simulink model "testcontroller"  (R2024b)
settings: Solver=VariableStepAuto  StartTime=0.0  StopTime=100.0  RelTol=1e-3
undefined symbols (not defined in the file): f, LF
libraries: slpidlib x6, instrumentseriallib x2, instrumentlib x1
settings Model: Creator=PC  LastModifiedBy=PC

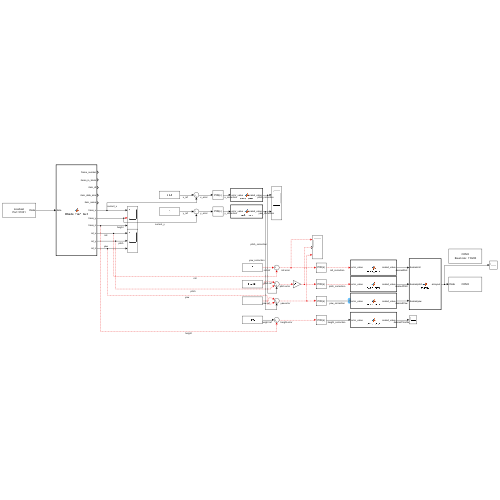
[thumbnail: Simulink's stored preview of the top-level diagram]
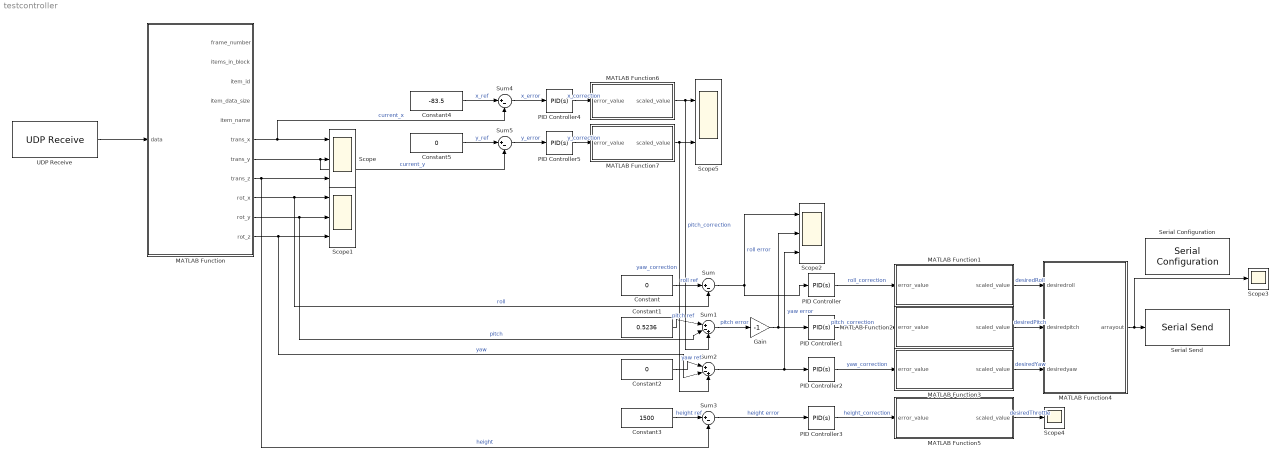
== system testcontroller ==
  Constant : Constant  Value=0
  Constant1 : Constant  Value=0.5236
  Constant2 : Constant  Value=0
  Constant3 : Constant  Value=1500
  Constant4 : Constant  Value=-83.5
  Constant5 : Constant  Value=0
  Gain : Gain  Gain=-1
  MATLAB Function : MATLAB Function  TreatAsAtomicUnit=on
  MATLAB Function1 : MATLAB Function  TreatAsAtomicUnit=on
  MATLAB Function2 : MATLAB Function  TreatAsAtomicUnit=on
  MATLAB Function3 : MATLAB Function  TreatAsAtomicUnit=on
  MATLAB Function4 : MATLAB Function  TreatAsAtomicUnit=on
  MATLAB Function5 : MATLAB Function  TreatAsAtomicUnit=on
  MATLAB Function6 : MATLAB Function  TreatAsAtomicUnit=on
  MATLAB Function7 : MATLAB Function  TreatAsAtomicUnit=on
  PID Controller{,1..5} (6 alike) : slpidlib/PID Controller  Controller=PID  Form=Parallel  TimeDomain=Continuous-time  UseExternalTs=off  SampleTime=-1  IntegratorMethod=Forward Euler  FilterMethod=Forward Euler  ControllerParametersSource=internal  P=1  I=0  UseKiTs=off  D=0  UseExternalDerivativeSource=off  N=100  UseFilter=on  TunerSelectOption=Transfer Function Based (PID Tuner App)  InitialConditionSource=internal  InitialConditionForIntegrator=0  InitialConditionForFilter=0  DifferentiatorICPrevScaledInput=0  ExternalReset=none  TrackingMode=off  Kt=1  LimitOutput=off  SatLimitsSource=internal  UpperSaturationLimit=inf  LowerSaturationLimit=-inf  LinearizeAsGain=on  AntiWindupMode=none  Kb=1  LimitIntegrator=off  UpperIntegratorSaturationLimit=inf  LowerIntegratorSaturationLimit=-inf  POutMin=[]  POutMax=[]  IOutMin=[]  IOutMax=[]  DOutMin=[]  DOutMax=[]  NOutMin=[]  NOutMax=[]  SumOutMin=[]  SumOutMax=[]  SaturationOutMin=[]  SaturationOutMax=[]  PParamMin=[]  PParamMax=[]  IParamMin=[]  IParamMax=[]  DParamMin=[]  DParamMax=[]  NParamMin=[]  NParamMax=[]  KbParamMin=[]  KbParamMax=[]  KtParamMin=[]  KtParamMax=[]  KbOutMin=[]  KbOutMax=[]  KtOutMin=[]  KtOutMax=[]  IntegratorOutMin=[]  IntegratorOutMax=[]  FilterOutMin=[]  FilterOutMax=[]  SumI1OutMin=[]  SumI1OutMax=[]  SumI2OutMin=[]  SumI2OutMax=[]  SumI3OutMin=[]  SumI3OutMax=[]  SumI4OutMin=[]  SumI4OutMax=[]  SumDOutMin=[]  SumDOutMax=[]  DifferentiatorOutMin=[]  DifferentiatorOutMax=[]  FilterDiffOutCoefMin=[]  FilterDiffOutCoefMax=[]  ReciprocalOutMin=[]  ReciprocalOutMax=[]  SumDenOutMin=[]  SumDenOutMax=[]  SumNumOutMin=[]  SumNumOutMax=[]  DivideOutMin=[]  DivideOutMax=[]  UdiffTsProdOutMin=[]  UdiffTsProdOutMax=[]  NTsProdOutMin=[]  NTsProdOutMax=[]  UintegralTsProdOutMin=[]  UintegralTsProdOutMax=[]  UngainTsProdOutMin=[]  UngainTsProdOutMax=[]  ClampingZeroOutDataTypeStr=Inherit: Inherit via back propagation  ClampingZeroOutMin=[]  ClampingZeroOutMax=[]  FilterDenConstantOutDataTypeStr=Inherit: Inherit via back propagation  FilterDenConstantOutMin=[]  FilterDenConstantOutMax=[]  PCopyOutDataTypeStr=Inherit: Inherit via back propagation  PCopyOutMin=[]  PCopyOutMax=[]  NCopyOutDataTypeStr=Inherit: Inherit via back propagation  NCopyOutMin=[]  NCopyOutMax=[]  IntegratorContinuousStateAttributes=''  IntegratorStateMustResolveToSignalObject=off  IntegratorRTWStateStorageClass=Auto  FilterContinuousStateAttributes=''  FilterStateMustResolveToSignalObject=off  FilterRTWStateStorageClass=Auto  ParallelPVariant=InternalParameters  IdealPVariant=Disabled  IVariant=InternalParameters  DVariant=InternalParameters  IntegratorVariant=Continuous  SatVariant=Disabled  AWVariant=Passthrough  PCopyVariant=Disabled  TRVariant=Disabled  FdbkBlocksVariant=Forward  IdealPFdbkVariant=Disabled  SatFdbkVariant=Disabled  DerivativeFilterVariant=ContFilter  NVariant=InternalParameters  NCopyVariant=Disabled  FilterICVariant=InternalICsFilter  IntegratorICVariant=InternalICs  ExternalResetVariant=Disabled  TRSumVariant=Passthrough  SumFdbkVariant=Disabled  SumVariant=Sum_PID  TsampFilterVariant=InternalTs  TsampNgainVariant=Passthrough  TsampIntegralVariant=Disabled_SignalSpec  ExternalSaturationOutDataTypeStr=Inherit: Same as second input  DerivativeSourceVariant=ErrorSignal  PreIntVariant=InternalPreInt
  Scope : Scope  NumInputPorts=3
  Scope1 : Scope  NumInputPorts=3
  Scope2 : Scope  NumInputPorts=3
  Scope3 : Scope
  Scope4 : Scope
  Scope5 : Scope  NumInputPorts=2
  Serial Configuration : instrumentseriallib/Serial Configuration  Priority=-200000  PortSel=COM3  Port=COM3  ComPort=COM3  BaudRate=115200  DataBits=8  Parity=none  StopBits=1  ByteOrder=little-endian  FlowControl=none  Timeout=10  SimulateUsing=Interpreted execution  BlockInModel=on  aMode=1
  Serial Send : instrumentseriallib/Serial Send  Priority=1  PortSel=COM3  Port=COM3  ComPort=COM3  Header=[]  Terminator=LF ('\n')  CustomTerminator=[]  EnableBlockingMode=on  SimulateUsing=Interpreted execution  BlockInModel=on  aMode=1
  Sum{,3..5} (4 alike) : Sum  Inputs=|+-
  Sum1 : Sum  Inputs=|+-+
  Sum2 : Sum  Inputs=|+-+
  UDP Receive : instrumentlib/UDP Receive  LocalAddress=localhost  LocalPort=51001  EnablePortSharing=off  Host=localhost  Port=9090  GetLatestData=on  DataSize=[1024, 1]  DataType=uint8  ASCIIFormatting=%f,  Terminator=LF  CustomTerminator=10  ByteOrder=big-endian  EnableBlockingMode=on  Timeout=10  SampleTime=0.02  SimulateUsing=Interpreted execution
  wires:
  UDP Receive/1 -> MATLAB Function/1(data)
  MATLAB Function/7(trans_y) -> Sum5/2, Scope/2  "current_y"
  MATLAB Function/8(trans_z) -> Scope/3, Sum3/2  "height"
  MATLAB Function/9(rot_x) -> Scope1/1, Sum/2  "roll"
  MATLAB Function/10(rot_y) -> Scope1/2, Sum1/2  "pitch"
  MATLAB Function/11(rot_z) -> Scope1/3, Sum2/2  "yaw"
  Constant/1 -> Sum/1  "roll ref"
  Constant1/1 -> Sum1/1  "pitch ref"
  Constant2/1 -> Sum2/1  "yaw ref"
  Sum/1 -> PID Controller/1, Scope2/1  "roll error"
  Sum1/1 -> Gain/1  "pitch error"
  Sum2/1 -> PID Controller2/1, Scope2/3  "yaw error"
  PID Controller/1 -> MATLAB Function1/1(error_value)  "roll_correction"
  PID Controller1/1 -> MATLAB Function2/1(error_value)  "pitch_correction"
  PID Controller2/1 -> MATLAB Function3/1(error_value)  "yaw_correction"
  MATLAB Function3/1(scaled_value) -> MATLAB Function4/3(desiredyaw)  "desiredYaw"
  MATLAB Function1/1(scaled_value) -> MATLAB Function4/1(desiredroll)  "desiredRoll"
  MATLAB Function2/1(scaled_value) -> MATLAB Function4/2(desiredpitch)  "desiredPitch"
  MATLAB Function4/1(arrayout) -> Serial Send/1, Scope3/1
  Gain/1 -> Scope2/2, PID Controller1/1
  Constant3/1 -> Sum3/1  "height ref"
  Sum3/1 -> PID Controller3/1  "height error"
  MATLAB Function5/1(scaled_value) -> Scope4/1  "desiredThrottle"
  PID Controller3/1 -> MATLAB Function5/1(error_value)  "height_correction"
  Sum5/1 -> PID Controller5/1  "y_error"
  Sum4/1 -> PID Controller4/1  "x_error"
  Constant4/1 -> Sum4/1  "x_ref"
  Constant5/1 -> Sum5/1  "y_ref"
  MATLAB Function/6(trans_x) -> Sum4/2, Scope/1  "current_x"
  PID Controller4/1 -> MATLAB Function6/1(error_value)  "x_correction"
  PID Controller5/1 -> MATLAB Function7/1(error_value)  "y_correction"
  MATLAB Function6/1(scaled_value) -> Scope5/1, Sum1/3  "pitch_correction"
  MATLAB Function7/1(scaled_value) -> Scope5/2, Sum2/3  "yaw_correction"

== matlab function testcontroller/MATLAB Function1 ==
  data: error_value input; scaled_value output
function scaled_value = scale_error(error_value)
    % Define the original and target ranges
    a = -pi/2;
    b = pi/2;
    c = 500;
    d = 1500;

    % Apply the scaling formula
    scaled_value = c + ((error_value - a) * (d - c)) / (b - a);
end

== matlab function testcontroller/MATLAB Function ==
  data: data input; frame_number output; items_in_block output; item_id output; item_data_size output; item_name output; trans_x output; trans_y output; trans_z output; rot_x output; rot_y output; rot_z output
function [frame_number, items_in_block, item_id, item_data_size, item_name, ...
    trans_x, trans_y, trans_z, rot_x, rot_y, rot_z] = decode_vicon_data(data)
    % Define expected output sizes explicitly
    % Set up each output as an array with dimensions (1x1) or (8x1) as needed.

    % Initialize output arrays
    frame_number = zeros(1, 1, 'uint32');  % Explicitly scalar output
    items_in_block = zeros(1, 1, 'uint8');  % Explicitly scalar output
    item_id = zeros(1, 1, 'uint8');        % Explicitly scalar output
    item_data_size = zeros(1, 1, 'uint16'); % Explicitly scalar output
    item_name = zeros(24, 1, 'uint8');     % 24 bytes for item name, uint8 array
    trans_x = zeros(1, 1, 'double');       % Scalar, double
    trans_y = zeros(1, 1, 'double');       % Scalar, double
    trans_z = zeros(1, 1, 'double');       % Scalar, double
    rot_x = zeros(1, 1, 'double');         % Scalar, double
    rot_y = zeros(1, 1, 'double');         % Scalar, double
    rot_z = zeros(1, 1, 'double');         % Scalar, double

    % Frame Number (4 bytes, uint32), scalar
    frame_number = typecast(data(1:4), 'uint32');
    
    % ItemsInBlock (1 byte, uint8)
    items_in_block = uint8(data(5));  % Scalar uint8
    
    % Item ID (1 byte, uint8) (0 for object data)
    item_id = uint8(data(6));  % Scalar uint8
    
    % Item Data Size (2 bytes, uint16)
    item_data_size = typecast(data(7:8), 'uint16');  % Scalar uint16
    
    % Item Name (24 bytes, uint8) converted from char
    item_name = uint8(data(9:32));  % Cast to uint8 (ASCII values of characters)
    
    % Translation (TransX, TransY, TransZ) - 8 bytes each (double)
    trans_x = typecast(data(33:40), 'double');
    trans_y = typecast(data(41:48), 'double');
    trans_z = typecast(data(49:56), 'double');
    
    % Rotation (RotX, RotY, RotZ) - 8 bytes each (double)
    rot_x = typecast(data(57:64), 'double');
    rot_y = typecast(data(65:72), 'double');
    rot_z = typecast(data(73:80), 'double');
end

== matlab function testcontroller/MATLAB Function2 ==
  data: error_value input; scaled_value output
function scaled_value = scale_error(error_value)
    % Define the original and target ranges
    a = -pi/2;
    b = pi/2;
    c = 500;
    d = 1500;

    % Apply the scaling formula
    scaled_value = c + ((error_value - a) * (d - c)) / (b - a);
end

== matlab function testcontroller/MATLAB Function3 ==
  data: error_value input; scaled_value output
function scaled_value = scale_error(error_value)
    % Define the original and target ranges
    a = -pi;
    b = pi;
    c = 500;
    d = 1500;

    % Apply the scaling formula
    scaled_value = c + ((error_value - a) * (d - c)) / (b - a);
end

== matlab function testcontroller/MATLAB Function4 ==
  data: desiredroll input; desiredpitch input; arrayout output; desiredyaw input
% MATLAB Function code
function arrayout = toarray(desiredroll, desiredpitch, desiredyaw)
    % Cast each input value to int32
    desiredroll = int16(desiredroll);  
    desiredpitch = int16(desiredpitch);  
    desiredyaw = int16(desiredyaw);  
    
    % Store the values in an array
    arrayout = [desiredroll, desiredpitch, desiredyaw];
    
    % Print the values as comma-separated integers with newline
    %fprintf('%d,%d,%d\n', arrayout(1), arrayout(2), arrayout(3));
end

== matlab function testcontroller/MATLAB Function5 ==
  data: error_value input; scaled_value output
function scaled_value = scale_error(error_value)
    % Define the original and target ranges
    a = -1000;
    b = 1000;
    c = 500;
    d = 1500;

    % Apply the scaling formula
    scaled_value = c + ((error_value - a) * (d - c)) / (b - a);
end

== matlab function testcontroller/MATLAB Function6 ==
  data: error_value input; scaled_value output
function scaled_value = scale_error(error_value)
    % Define the original and target ranges
    a = -1000;
    b = 1000;
    c = -pi/6;
    d = pi/6;

    % Apply the scaling formula
    scaled_value = c + ((error_value - a) * (d - c)) / (b - a);
end

== matlab function testcontroller/MATLAB Function7 ==
  data: error_value input; scaled_value output
function scaled_value = scale_error(error_value)
    % Define the original and target ranges
    a = -1000;
    b = 1000;
    c = -pi/6;
    d = pi/6;

    % Apply the scaling formula
    scaled_value = c + ((error_value - a) * (d - c)) / (b - a);
end
